simulink model "C28x_Vehicle_Dynamics_"  (Simulink 6.5)
settings: Solver=FixedStepDiscrete  StartTime=0.0  StopTime=inf  RelTol=1e-3
values from neighbouring files (symbols this model uses):
  x = single(get(hObject,'Value'))    [AM.m]
undefined symbols (not defined in the file or in its folder): DiscIntNeverNeededParam
libraries: c281xdspchiplib x2, simulink x1, c2000tgtpreflib x1
settings Model: Creator=Dell  LastModifiedBy=Dell  ProdHWDeviceType=TI C2000
settings DataIOCC: SaveOutput=off  SaveTime=off
settings OptimizationCC: OptimizeModelRefInitCode=on  LifeSpan=1
settings HardwareCC: ProdBitPerChar=16  ProdBitPerInt=16  ProdIntDivRoundTo=Zero  ProdEndianess=LittleEndian  ProdWordSize=16  ProdHWDeviceType=TI C2000  TargetHWDeviceType=32-bit Generic
settings RTWCC: SystemTargetFile=ti_c2000_ert.tlc  TemplateMakefile=ti_c2000_ert.tmf  Description=Embedded Target for TI C2000 DSP (ERT)  ProcessScript=ti_c2000_ert_make_rtw_hook
settings CodeAppCC: IgnoreCustomStorageClasses=off
settings STFCustomTargetCC: TargetFcnLib=ansi_tfl_tmw.mat  GenFloatMathFcnCalls=ANSI_C  ModelReferenceCompliant=off  CombineOutputUpdateFcns=on  ERTCustomFileBanners=on  SupportContinuousTime=off  SupportNonInlinedSFcns=off  SystemTargetFile=ti_c2000_ert.tlc
settings ERTTargetCC: TargetFcnLib=ansi_tfl_tmw.mat  GenFloatMathFcnCalls=ANSI_C  ModelReferenceCompliant=off  InlinedParameterPlacement=NonHierarchical  ERTCustomFileTemplate=example_file_process.tlc

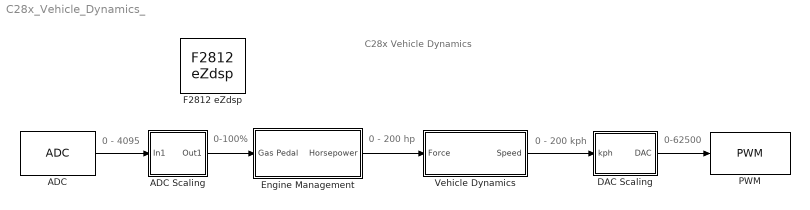
== system C28x_Vehicle_Dynamics_ ==
  note: 0 - 200 kph
  note: C28x Vehicle Dynamics
  note: 0 - 200 hp
  note: 0 - 4095
  note: 0-100%
  note: 0-62500
  " DAC Scaling" : Subsystem
  ADC : c281xdspchiplib/ADC  useModule=A  useMode=Sequential  sourceSOC=Software  Ts=0.001  dType=uint16  postInterrupt=off  numConversionsSingle=1  numConversionsDouble=1  conv0=ADCINB0  conv1=ADCINB1  conv2=ADCINB2  conv3=ADCINB3  conv4=ADCINA4  conv5=ADCINA5  conv6=ADCINB6  conv7=ADCINA7  conv8=ADCINB0  conv9=ADCINB1  conv10=ADCINB2  conv11=ADCINB3  conv12=ADCINB4  conv13=ADCINB5  conv14=ADCINB6  conv15=ADCINB7  convAB0=ADCINA0 and ADCINB0  convAB1=ADCINA1 and ADCINB1  convAB2=ADCINA5 and ADCINB5  convAB3=ADCINA1 and ADCINB1  convAB4=ADCINA1 and ADCINB1  convAB5=ADCINA1 and ADCINB1  convAB6=ADCINA1 and ADCINB1  convAB7=ADCINA1 and ADCINB1  convA0=ADCINA0  convA1=ADCINA1  convA2=ADCINA2  convA3=ADCINA3  convA4=ADCINA4  convA5=ADCINA5  convA6=ADCINA6  convA7=ADCINA7  convB0=ADCINB0  convB1=ADCINB1  convB2=ADCINB2  convB3=ADCINB3  convB4=ADCINB4  convB5=ADCINB5  convB6=ADCINB6  convB7=ADCINB7  c28xmultiPort=off
  ADC Scaling : Subsystem
  Engine Management : Subsystem
  F2812 eZdsp : c2000tgtpreflib/F2812 eZdsp  Tag=C2000 TARGET PREFERENCES BLOCK  SystemSampleTime=-1
  PWM : c281xdspchiplib/PWM  useModule=A  timerSource=Input port  timerPeriod=37500  waveformType=Asymmetric  periodUnits=Clock cycles  unit1Status=on  unit1Source=Specify via dialog  unit1Value=62500  unit2Status=off  unit2Source=Specify via dialog  unit2Value=18500  unit3Status=off  unit3Source=Specify via dialog  unit3Value=18500  dutyCycleUnits=Clock cycles  logicSource=Specify via dialog  unit1_1Logic=Active high  unit1_2Logic=Active low  unit2_1Logic=Active high  unit2_2Logic=Active low  unit3_1Logic=Active high  unit3_2Logic=Active low  enableDeadband1=off  enableDeadband2=off  enableDeadband3=off  deadbandPrescaler=1  deadbandPeriodSource=Specify via dialog  deadbandPeriod=1  adcstartEvent=None
  "Vehicle Dynamics " : Subsystem
  wires:
  "Vehicle Dynamics "/1(Speed) -> " DAC Scaling"/1(kph)
  Engine Management/1(Horsepower) -> "Vehicle Dynamics "/1(Force)
  ADC Scaling/1(Out1) -> Engine Management/1(Gas Pedal)
  " DAC Scaling"/1(DAC) -> PWM/1
  ADC/1 -> ADC Scaling/1(In1)

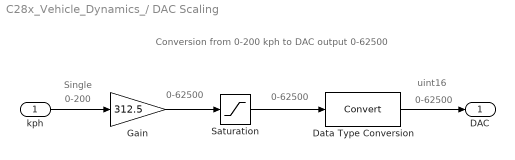
== system C28x_Vehicle_Dynamics_/ DAC Scaling ==
  note: 0-200
  note: 0-62500
  note: 0-62500
  note: Conversion from 0-200 kph to DAC output 0-62500
  note: Single
  note: uint16
  note: 0-62500
  kph : Inport
  Data Type Conversion : DataTypeConversion  OutDataTypeMode=uint16
  Gain : Gain  Gain=312.5
  Saturation : Saturate  UpperLimit=62500  LowerLimit=0
  DAC : Outport
  wires:
  kph/1 -> Gain/1
  Saturation/1 -> Data Type Conversion/1
  Gain/1 -> Saturation/1
  Data Type Conversion/1 -> DAC/1

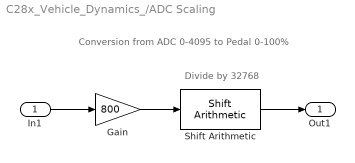
== system C28x_Vehicle_Dynamics_/ADC Scaling ==
  note: Divide by 32768
  note: Conversion from ADC 0-4095 to Pedal 0-100%
  In1 : Inport
  Gain : Gain  Gain=800  OutDataTypeMode=Specify via dialog  OutDataType=uint(32)
  Shift Arithmetic : simulink/Logic and Bit Operations/Shift Arithmetic  SystemSampleTime=-1  nBitShiftRight=15  nBinPtShiftRight=0
  Out1 : Outport
  wires:
  In1/1 -> Gain/1
  Gain/1 -> Shift Arithmetic/1
  Shift Arithmetic/1 -> Out1/1

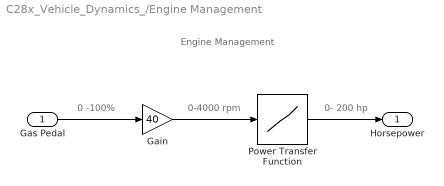
== system C28x_Vehicle_Dynamics_/Engine Management ==
  note: 0-4000 rpm
  note: 0 -100%
  note: 0- 200 hp
  note: Engine Management
  Gas Pedal : Inport
  Gain : Gain  Gain=40  ParameterDataTypeMode=Specify via dialog  ParameterDataType=uint(16)
  Power Transfer Function : Lookup  InputValues=uint16([0,500,1000,1500,2000,2500,3000,3500,4000]);  OutputValues=uint16([40,80,120,154,176,191,200,180,160]);  LookUpMeth=Interpolation-Extrapolation  OutDataTypeMode=uint16  OutDataType=sfix(16)  OutScaling=2^0  SampleTime=-1  LUTDesignTableMode=Redesign Table  LUTDesignDataSource=Block Dialog  LUTDesignFunctionName=sqrt(x)  LUTDesignUseExistingBP=on  LUTDesignRelError=0.01  LUTDesignAbsError=1e-6  SaturateOnIntegerOverflow=off  RndMeth=Floor
      settings: LockScale=off
  Horsepower : Outport
  wires:
  Gas Pedal/1 -> Gain/1
  Gain/1 -> Power Transfer Function/1
  Power Transfer Function/1 -> Horsepower/1

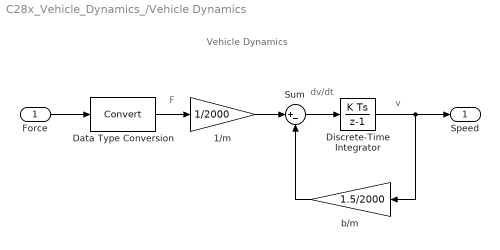
== system C28x_Vehicle_Dynamics_/Vehicle Dynamics  ==
  note: Vehicle Dynamics
  note: dv/dt
  note: v
  note: F
  Force : Inport
  1/m : Gain  Gain=1/2000
  Data Type Conversion : DataTypeConversion  OutDataTypeMode=single
  Discrete-Time Integrator : DiscreteIntegrator  ICPrevOutput=DiscIntNeverNeededParam  ICPrevScaledInput=DiscIntNeverNeededParam
  Sum : Sum  Inputs=|+-
  b/m : Gain  Orientation=left  Gain=1.5/2000
  Speed : Outport
  wires:
  Force/1 -> Data Type Conversion/1
  1/m/1 -> Sum/1
  Discrete-Time Integrator/1 -> Speed/1, b/m/1
  Sum/1 -> Discrete-Time Integrator/1
  b/m/1 -> Sum/2
  Data Type Conversion/1 -> 1/m/1
